simulink model "ME190_HW2_Justin_Garcia_StepInput"  (R2016b)
settings: Solver=ode5  StartTime=0.0  StopTime=10.0  FixedStep=.01  RelTol=1e-3
values from neighbouring files (symbols this model uses):
  Kd = 7    [ME190_HW2_Justin_Garcia.m]
  Ki = 0    [ME190_HW2_Justin_Garcia.m]
  Kp = 100    [ME190_HW2_Justin_Garcia.m]
  m = .2    (= 0.2)    [ME190_HW2_Justin_Garcia.m]
settings Model: Creator=Mac  LastModifiedBy=Mac

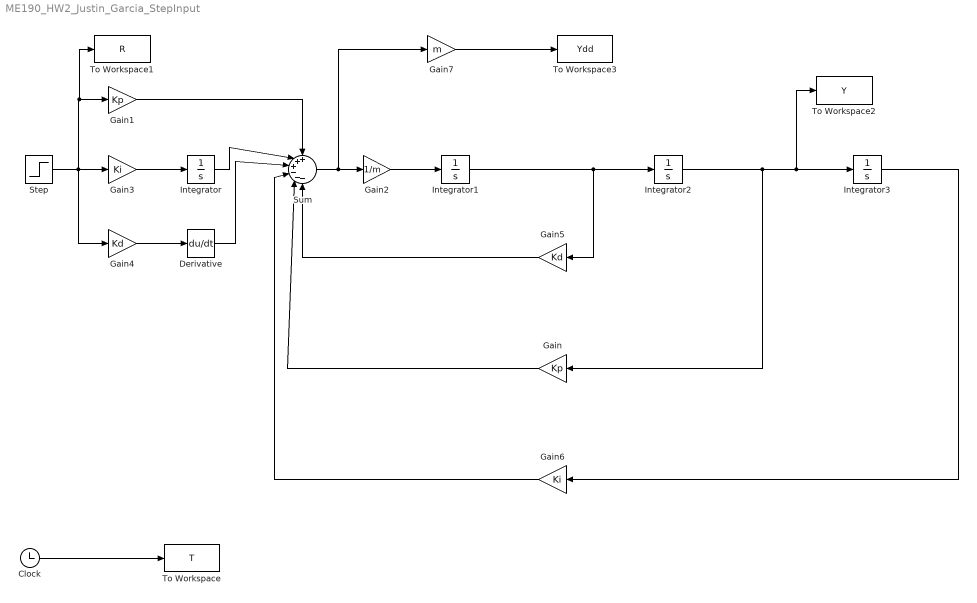
== system ME190_HW2_Justin_Garcia_StepInput ==
  Clock : Clock
  Derivative : Derivative
  Gain : Gain  Gain=Kp
  Gain1 : Gain  Gain=Kp
  Gain2 : Gain  Gain=1/m
  Gain3 : Gain  Gain=Ki
  Gain4 : Gain  Gain=Kd
  Gain5 : Gain  Gain=Kd
  Gain6 : Gain  Gain=Ki
  Gain7 : Gain  Gain=m
  Integrator{,1..3} (4 alike) : Integrator
  Step : Step  SampleTime=0
  Sum : Sum  Inputs=+++---
  To Workspace : ToWorkspace  VariableName=T  SampleTime=-1
  To Workspace1 : ToWorkspace  VariableName=R  SampleTime=-1
  To Workspace2 : ToWorkspace  VariableName=Y  SampleTime=-1
  To Workspace3 : ToWorkspace  VariableName=Ydd  SampleTime=-1
  wires:
  Gain2/1 -> Integrator1/1
  Integrator1/1 -> Gain5/1, Integrator2/1
  Integrator2/1 -> Gain/1, To Workspace2/1, Integrator3/1
  Integrator3/1 -> Gain6/1
  Step/1 -> Gain4/1, To Workspace1/1, Gain1/1, Gain3/1
  Gain3/1 -> Integrator/1
  Gain4/1 -> Derivative/1
  Gain1/1 -> Sum/1
  Integrator/1 -> Sum/2
  Derivative/1 -> Sum/3
  Gain5/1 -> Sum/6
  Gain/1 -> Sum/5
  Gain6/1 -> Sum/4
  Clock/1 -> To Workspace/1
  Sum/1 -> Gain7/1, Gain2/1
  Gain7/1 -> To Workspace3/1
